simulink model "IO135_test"  (R2022b)
settings: Solver=FixedStepAuto  StartTime=0.0  StopTime=Inf  RelTol=1e-3
model workspace (MAT data in the model file):
  sos1 = Simulink.Parameter
  sos1.Value = [1  0  0  1  0  0; 1  0  0  1  0  0; 1  0  0  1  0  0; 1  0  0  1  0  0]
  sos1.DataType = 'double'
  sos1.Complexity = 'real'
  sos1.Dimensions = [4 6]
  sos2 = Simulink.Parameter
  sos2.Value = [0  0  0  1  0  0; 1  0  0  1  0  0; 1  0  0  1  0  0; 1  0  0  1  0  0]
  sos2.DataType = 'double'
  sos2.Complexity = 'real'
  sos2.Dimensions = [4 6]
  stdev = Simulink.Parameter
  stdev.Value = 0.2
  stdev.DataType = 'double'
  stdev.Complexity = 'real'
  stdev.Dimensions = [1 1]
libraries: speedgoatlib_IO135 x3, slrealtimeloglib x2, SG_library x1
settings Model: LastModifiedBy=mavolery
settings SolverCC: ConcurrentTasks=on  PositivePriorityOrder=on
settings OptimizationCC: BlockReduction=off  BooleanDataType=off  DefaultParameterBehavior=Inlined  OptimizeBlockIOStorage=off
settings DebuggingCC: SaveWithParameterizedLinksMsg=none  UnderspecifiedInitializationDetection=Classic  MergeDetectMultiDrivingBlocksExec=none  SignalResolutionControl=TryResolveAllWithWarning  InheritedTsInSrcMsg=none  TasksWithSamePriorityMsg=none
settings HardwareCC: ProdBitPerLong=64  ProdLongLongMode=on  ProdHWDeviceType=Intel->x86-64 (Linux 64)
settings ModelReferenceCC: EnableRefExpFcnMdlSchedulingChecks=on  PropagateSignalLabelsOutOfModel=off
settings RTWCC: Description=Simulink Real-Time  SystemTargetFile=slrealtime.tlc  TemplateMakefile=slrealtime_default_tmf  RTWVerbose=off  Toolchain=Simulink Real-Time Toolchain  BuildConfiguration=Faster Runs  CodeExecutionProfiling=on  TargetLang=C++

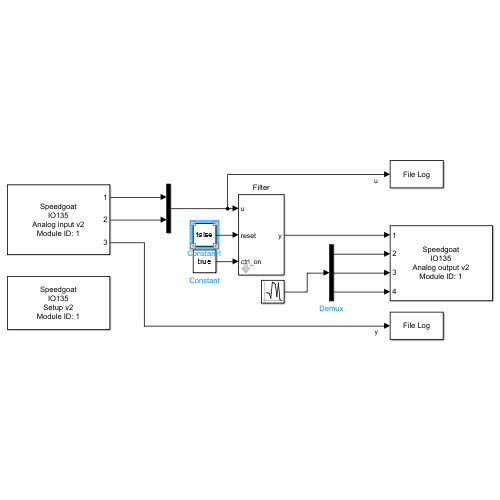
[thumbnail: Simulink's stored preview of the top-level diagram]
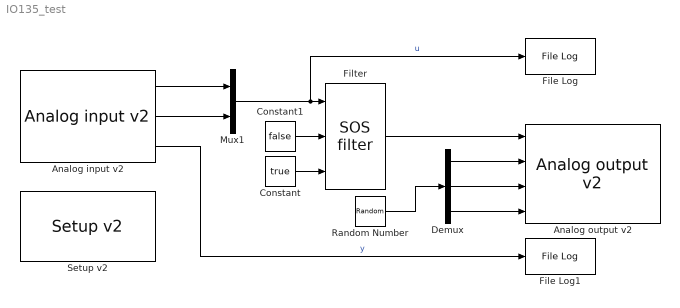
== system IO135_test ==
  "Analog input v2 " : speedgoatlib_IO135/Analog input v2   parModuleId=1  parSampleTime=-1  parPciSlot=-1  parAdcChannels=[1 2 3]  parAdcVoltageRange=[2 2 2 2]  parAdcOversamplRate=[1 1 1 1]  parAdcContSampling=0  parAdcDmaEnable=0  parAdcActiveDmaDevices=[1 1 1 1]  parAdcFrameSize=100
      settings: SourceProductName=Simulink Real-Time: Speedgoat I/O Blockset
  "Analog output v2 " : speedgoatlib_IO135/Analog output v2   parModuleId=1  parSampleTime=-1  parPciSlot=-1  parDacChannels=[1 2 3 4]  parDacVoltageRange=[5 5 5 5 5 5 5 5 5 5 5 5 5 5 5 5]  parDacInitValues=[0 0 0 0]  parDacReset=[1 1 1 1]  parDacSyncOut=1  parDacDmaEnable=0  parDacActiveDmaDevices=[1 1 1 1]  parDacDmaLatency=2  parDacFrameSize=100
      settings: SourceProductName=Simulink Real-Time: Speedgoat I/O Blockset
  Constant : Constant  Value=true  SampleTime=-1
  Constant1 : Constant  Value=false  SampleTime=-1
  Demux : Demux  Outputs=3
  File Log : slrealtimeloglib/File Log  decimation=1  inputProcessing=Elements as channels (sample based)
  File Log1 : slrealtimeloglib/File Log  decimation=1  inputProcessing=Elements as channels (sample based)
  Filter : SG_library/Source elements/SOS filter  sos1=sos1  sos2=sos2  limit_ctrl=10  ts=-1
      settings: SourceProductName=Custom Speedgoat implementations
  Mux1 : Mux  Inputs=2
  Random Number : RandomNumber  Variance=stdev  Seed=0:2  SampleTime=5e-05
  "Setup v2 " : speedgoatlib_IO135/Setup v2   parPciSlot=-1  parModuleId=1  parInterModuleSync=None  parConvClockBaseRate=20MHz  parConvClock1Divider=20000  parConvClock2Divider=20000  parFrameTriggerEnable=off  parFrameTriggerDivider=10  parConvClock1BaseRate=1  parConvClock2BaseRate=1  parFrameTriggerClock=1  parAdcChannels=1:3  parAdcRange1=+-10V  parAdcRange2=+-10V  parAdcRange3=+-10V  parAdcRange4=+-10V  parAdcVoltageRange=[2 2 2 2]  parAdcOversampling1=None  parAdcOversampling2=None  parAdcOversampling3=None  parAdcOversampling4=None  parAdcOversamplRate=[1 1 1 1]  parAdcAutoCorrection=on  parAdcContSampling=off  parAdcDmaEnable=off  parAdcDmaClock=Clock 1  parAdcFrameSize_=100  parAdcSampleTime_=-1  parAdcActiveDmaDevices=[1 1 1 1]  parAdcFrameTriggerEnable=0  parAdcFrameSize=100  parAdcSampleTime=0.1  parDacChannels=1:4  parDacInitValues=0  parDacReset=1  parDacRange1=+-10V  parDacRange2=+-10V  parDacRange3=+-10V  parDacRange4=+-10V  parDacRange5=+-10V  parDacRange6=+-10V  parDacRange7=+-10V  parDacRange8=+-10V  parDacRange9=+-10V  parDacRange10=+-10V  parDacRange11=+-10V  parDacRange12=+-10V  parDacRange13=+-10V  parDacRange14=+-10V  parDacRange15=+-10V  parDacRange16=+-10V  parDacVoltageRange=[5 5 5 5 5 5 5 5 5 5 5 5 5 5 5 5]  parDacAutoCorrection=on  parDacSyncOut=on  parDacDmaEnable=off  parDacDmaLatency=Until next frame  parDacDmaClock=Clock 1  parDacFrameSize_=100  parDacSampleTime_=-1  parDacActiveDmaDevices=[1 1 1 1]  parDacFrameTriggerEnable=0  parDacFrameSize=100  parDacSampleTime=0.1  parDoChannels=[]  parDoInitValues=0  parDoReset=1  parDiChannels=[]  parDiDebounceEnable=off  parDiDebounceTime=0  parDiDebounceValue=0  parDioPullRefFront=Pull-up 3.3V  parDioPullRefRear=Floating
      settings: SourceProductName=Simulink Real-Time: Speedgoat I/O Blockset
  wires:
  Filter/1 -> "Analog output v2 "/1
  Mux1/1 -> File Log/1, Filter/1  "u"
  "Analog input v2 "/1 -> Mux1/1
  "Analog input v2 "/2 -> Mux1/2
  "Analog input v2 "/3 -> File Log1/1  "y"
  Constant/1 -> Filter/3
  Constant1/1 -> Filter/2
  Demux/2 -> "Analog output v2 "/3
  Demux/1 -> "Analog output v2 "/2
  Demux/3 -> "Analog output v2 "/4
  Random Number/1 -> Demux/1
